simulink model "Ejercicio22_27_02_17"  (R2013a)
settings: Solver=ode45  StartTime=0.0  StopTime=10.0  RelTol=1e-3
settings Model: Creator=Miguel  LastModifiedBy=Miguel

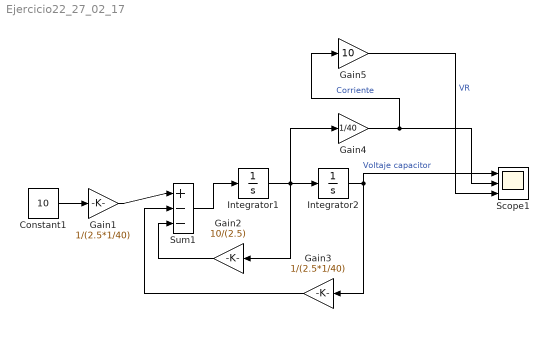
== system Ejercicio22_27_02_17 ==
  Constant1 : Constant  Value=10
  Gain1 : Gain  Gain=1/(2.5*1/40)
  Gain2 : Gain  Gain=10/(2.5)
  Gain3 : Gain  Gain=1/(2.5*1/40)
  Gain4 : Gain  Gain=1/40
  Gain5 : Gain  Gain=10
  Integrator1 : Integrator
  Integrator2 : Integrator  InitialCondition=8
  Scope1 : Scope  NumInputPorts=3
      settings: ShowLegends=on  YMin=-5~-5~-5  YMax=5~5~5
  Sum1 : Sum  Inputs=|+--
  wires:
  Integrator1/1 -> Gain4/1, Gain2/1, Integrator2/1
  Integrator2/1 -> Scope1/1, Gain3/1  "Voltaje capacitor"
  Sum1/1 -> Integrator1/1
  Gain2/1 -> Sum1/3
  Gain3/1 -> Sum1/2
  Constant1/1 -> Gain1/1
  Gain1/1 -> Sum1/1
  Gain4/1 -> Gain5/1, Scope1/2  "Corriente"
  Gain5/1 -> Scope1/3  "VR"
